simulink model "sim_GPID_LOS"  (R2017a)
settings: Solver=FixedStepAuto  StartTime=0.0  StopTime=inf  FixedStep=0.01  RelTol=1e-3
values from neighbouring files (symbols this model uses):
  trial_params = sim_params(i)    [exec_sim_main.m]
undefined symbols (not defined in the file or in its folder): update_wrap
libraries: simulink x3, emily x1
settings Model: Creator=mitchallain  LastModifiedBy=mitchallain
settings DataIOCC: SaveOutput=off  SaveTime=off

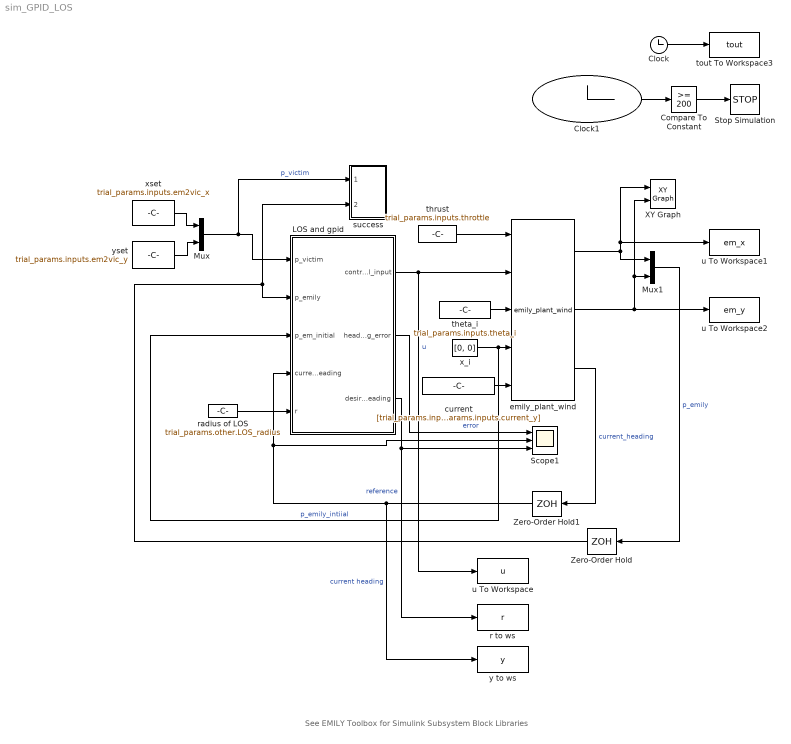
== system sim_GPID_LOS ==
  note: See EMILY Toolbox for Simulink Subsystem Block Libraries
  Clock : Clock
  Clock1 : Clock
  Compare To Constant : simulink/Logic and Bit Operations/Compare To Constant  relop=>=  const=200  OutDataTypeStr=boolean
  LOS and gpid : Subsystem
  Mux : Mux  Inputs=2
  Mux1 : Mux  Inputs=2
  Scope1 : Scope  NumInputPorts=3
  Stop Simulation : Stop
  XY Graph : simulink/Sinks/XY Graph  xmin=-50  xmax=50  ymin=-50  ymax=50  st=-1
  Zero-Order Hold : ZeroOrderHold  SampleTime=0.2
  Zero-Order Hold1 : ZeroOrderHold  SampleTime=0.2
  current : Constant  Value=[trial_params.inputs.current_x, trial_params.inputs.current_y]
  emily_plant_wind : emily/emily_plant_wind
      settings: SourceProductName=EMILY Toolbox
  r to ws : ToWorkspace  VariableName=r  SampleTime=0.2
  radius of LOS : Constant  Value=trial_params.other.LOS_radius
  success : Subsystem  AncestorBlock=emily/success
  theta_i : Constant  Value=trial_params.inputs.theta_i
  thrust : Constant  Value=trial_params.inputs.throttle
  tout To Workspace3 : ToWorkspace  VariableName=tout  SampleTime=0.2
  u To Workspace : ToWorkspace  VariableName=u  SampleTime=0.2
  u To Workspace1 : ToWorkspace  VariableName=em_x  SampleTime=0.2
  u To Workspace2 : ToWorkspace  VariableName=em_y  SampleTime=0.2
  x_i : Constant  Value=[0, 0]
  xset : Constant  Value=trial_params.inputs.em2vic_x
  y to ws : ToWorkspace  VariableName=y  SampleTime=0.2
  yset : Constant  Value=trial_params.inputs.em2vic_y
  wires:
  emily_plant_wind/1 -> XY Graph/1, u To Workspace1/1, Mux1/1
  Mux1/1 -> Zero-Order Hold/1  "p_emily"
  thrust/1 -> emily_plant_wind/1
  Mux/1 -> success/1(p_victim), LOS and gpid/1(p_victim)  "p_victim"
  theta_i/1 -> emily_plant_wind/3
  emily_plant_wind/3 -> Zero-Order Hold1/1  "current_heading"
  xset/1 -> Mux/1
  yset/1 -> Mux/2
  emily_plant_wind/2 -> XY Graph/2, Mux1/2, u To Workspace2/1
  LOS and gpid/2(heading_error) -> Scope1/1  "error"
  LOS and gpid/1(control_input) -> emily_plant_wind/2, u To Workspace/1  "u"
  LOS and gpid/3(desired_heading) -> Scope1/3, r to ws/1  "reference"
  x_i/1 -> LOS and gpid/3(p_em_initial), emily_plant_wind/4  "p_emily_intiial"
  radius of LOS/1 -> LOS and gpid/5(r)
  Zero-Order Hold/1 -> success/2(p_emily), LOS and gpid/2(p_emily)
  Zero-Order Hold1/1 -> y to ws/1, Scope1/2, LOS and gpid/4(current_heading)  "current heading"
  current/1 -> emily_plant_wind/5
  Clock/1 -> tout To Workspace3/1
  Clock1/1 -> Compare To Constant/1
  Compare To Constant/1 -> Stop Simulation/1

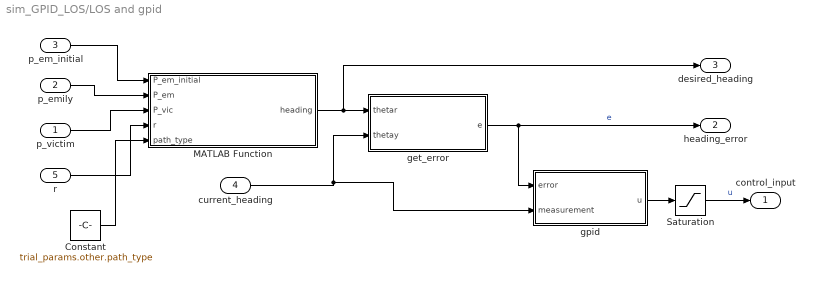
== system sim_GPID_LOS/LOS and gpid ==
  p_victim : Inport
  p_emily : Inport  Port=2
  p_em_initial : Inport  Port=3
  current_heading : Inport  Port=4
  r : Inport  Port=5
  Constant : Constant  Value=trial_params.other.path_type
  MATLAB Function : MATLAB Function  TreatAsAtomicUnit=on
  Saturation : Saturate  UpperLimit=pi/4  LowerLimit=-pi/4
  get_error : MATLAB Function  TreatAsAtomicUnit=on
  gpid : Subsystem
  control_input : Outport
  heading_error : Outport  Port=2
  desired_heading : Outport  Port=3
  wires:
  r/1 -> MATLAB Function/4(r)
  p_em_initial/1 -> MATLAB Function/1(P_em_initial)
  p_emily/1 -> MATLAB Function/2(P_em)
  p_victim/1 -> MATLAB Function/3(P_vic)
  current_heading/1 -> gpid/2(measurement), get_error/2(thetay)
  get_error/1(e) -> gpid/1(error), heading_error/1  "e"
  gpid/1(u) -> Saturation/1
  Saturation/1 -> control_input/1  "u"
  Constant/1 -> MATLAB Function/5(path_type)
  MATLAB Function/1(heading) -> get_error/1(thetar), desired_heading/1

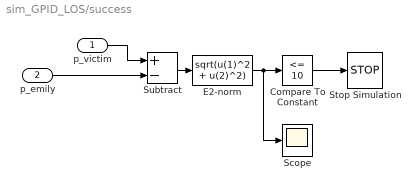
== system sim_GPID_LOS/success ==
  p_victim : Inport
  p_emily : Inport  Port=2
  Compare To Constant : simulink/Logic and Bit Operations/Compare To Constant  relop=<=  const=10  OutDataTypeStr=boolean
  E2-norm : Fcn  Expr=sqrt(u(1)^2 + u(2)^2)
  Scope : Scope
  Stop Simulation : Stop
  Subtract : Sum  Inputs=+-
  wires:
  Subtract/1 -> E2-norm/1
  E2-norm/1 -> Compare To Constant/1, Scope/1
  p_victim/1 -> Subtract/1
  Compare To Constant/1 -> Stop Simulation/1
  p_emily/1 -> Subtract/2

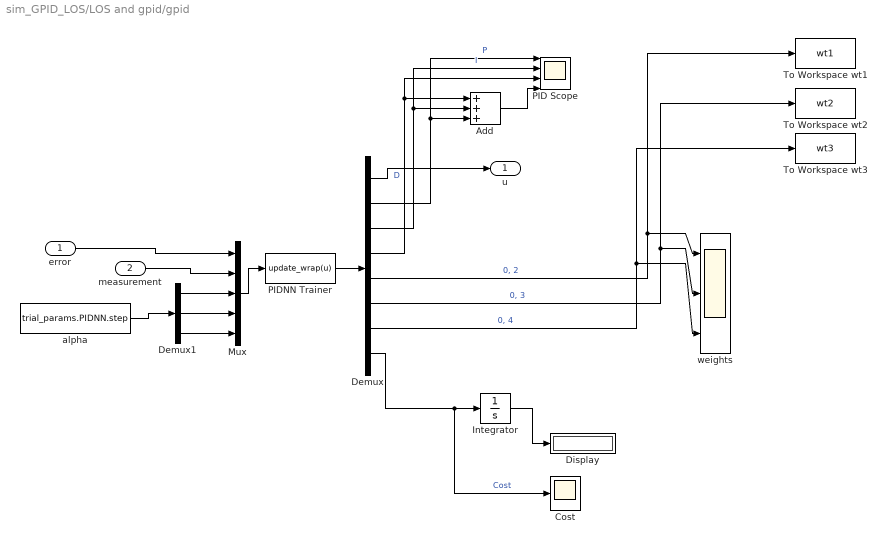
== system sim_GPID_LOS/LOS and gpid/gpid ==
  error : Inport
  measurement : Inport  Port=2
  Add : Sum  Inputs=+++
  Cost : Scope
  Demux : Demux  Outputs=8
  Demux1 : Demux  Outputs=3
  Display : Display
  Integrator : Integrator
  Mux : Mux  Inputs=5
  PID Scope : Scope  NumInputPorts=4
  PIDNN Trainer : MATLABFcn  MATLABFcn=update_wrap(u)  Output1D=off
  To Workspace wt1 : ToWorkspace  VariableName=wt1  SampleTime=-1
  To Workspace wt2 : ToWorkspace  VariableName=wt2  SampleTime=-1
  To Workspace wt3 : ToWorkspace  VariableName=wt3  SampleTime=-1
  alpha : Constant  Value=trial_params.PIDNN.step
  weights : Scope  NumInputPorts=3
  u : Outport
  wires:
  Integrator/1 -> Display/1
  Add/1 -> PID Scope/4
  alpha/1 -> Demux1/1
  Demux/7 -> To Workspace wt3/1, weights/3  "0, 4"
  Demux/6 -> To Workspace wt2/1, weights/2  "0, 3"
  measurement/1 -> Mux/2
  Demux/4 -> PID Scope/3, Add/1  "D"
  Demux/3 -> Add/2, PID Scope/2  "I"
  Mux/1 -> PIDNN Trainer/1
  error/1 -> Mux/1
  Demux/1 -> u/1
  PIDNN Trainer/1 -> Demux/1
  Demux/5 -> To Workspace wt1/1, weights/1  "0, 2"
  Demux/2 -> Add/3, PID Scope/1  "P"
  Demux/8 -> Cost/1, Integrator/1  "Cost"
  Demux1/1 -> Mux/3
  Demux1/2 -> Mux/4
  Demux1/3 -> Mux/5

== matlab function sim_GPID_LOS/LOS and gpid/get_error ==
  data: thetar input; e output; thetay input
function e  = get_error(thetar, thetay)
%UNTITLED Summary of this function goes here
%   FIX THIS MITCH
e = thetar - thetay;
e = mod((e + pi), 2*pi) - pi;
end

== matlab function sim_GPID_LOS/LOS and gpid/MATLAB Function ==
  data: P_em_initial input; heading output; P_em input; P_vic input; r input; path_type input
function heading  = straightpathLOS(P_em_initial, P_em, P_vic, r, path_type)
% This function computes the heading angle according to LOS geometric law
%   Assumes straight line path from initial location to victim
%   If two intersections are produced, the intersection with a higher
%   dispacement parameter (s) is chosen (i.e., farther along path)

% Args:
%   P_em_initial (2-vector): initial (x, y) location of EMILY
%   P_em (2-vector): current (x, y) location of EMILY
%   P_vic (2-vector): victim (x, y) location
%   r (float): radius for LOS control

% Returns:
%   heading: heading unit vector for EMILY in global frame
global trial_params;
% Compute vector from initial EMILY to victim in global frame
P_eiv = P_vic - P_em_initial;

% Compute desired path length and angle
d = norm(P_eiv);
path_angle = atan2(P_eiv(2), P_eiv(1));

% Compute vector from current EMILY to victim
P_ev = P_vic - P_em;

% Bearing is used to seed the fminsearch
bearing = atan2(P_ev(2), P_ev(1));

% Parameterized circle about emily
xLOS = @(phi) P_em(1) + r*cos(phi);
yLOS = @(phi) P_em(2) + r*sin(phi);

switch path_type
    case 1
        x = [P_em_initial(1) P_vic(1)/3  P_vic(1)*2/3  P_vic(1)]; %spline intersection pts
        y = [P_em_initial(2) P_vic(2)*2/3  P_vic(2)*2/3  P_vic(2)];
        pp = spline(x,y);
        path = @(s) ppval(pp,s);
        xy = @(param) (path(param(1)) - xLOS(param(2)))^2 + (path(param(1)) - yLOS(param(2)))^2;
        temp = fminsearch(@(param) xy(param), [P_em(1)+20*cos(bearing), bearing]);
        s_i = temp(1);
        phi_i = temp(2);
        P_es = [s_i - P_em(1); path(s_i) - P_em(2)];
        
    case 2
        x = [P_em_initial(1) P_vic(1)/3 P_vic(1)*2/3 P_vic(1)]; %spline intersection pts
        y = [P_em_initial(2) P_em_initial(2)*4/3 P_vic(2)/3  P_vic(2)];
        pp = spline(x,y);
        path = @(s) ppval(pp,s);
        xy = @(param) (path(param(1)) - xLOS(param(2)))^2 + (path(param(1)) - yLOS(param(2)))^2;
        temp = fminsearch(@(param) xy(param), [P_em(1)+20*cos(bearing), bearing]);
        s_i = temp(1);
        phi_i = temp(2);
        P_es = [s_i - P_em(1); path(s_i) - P_em(2)];
        
    case 3
        x = [P_em_initial(1) P_vic(1)/3 P_vic(1)*2/3 P_vic(1)]; %spline intersection pts
        y = [P_em_initial(2) P_vic(2)*2/3 P_em_initial(2)*4/3  P_vic(2)];
        pp = spline(x,y);
        path = @(s) ppval(pp,s);
        xy = @(param) (path(param(1)) - xLOS(param(2)))^2 + (path(param(1)) - yLOS(param(2)))^2;
        temp = fminsearch(@(param) xy(param), [P_em(1)+20*cos(bearing), bearing]);
        s_i = temp(1);
        phi_i = temp(2);
        P_es = [s_i - P_em(1); path(s_i) - P_em(2)];

    otherwise %'straight'
        xpath = @(s) P_em_initial(1) + s*cos(path_angle);
        ypath = @(s) P_em_initial(2) + s*sin(path_angle);
        xy = @(param) (xpath(param(1)) - xLOS(param(2)))^2 + (ypath(param(1)) - yLOS(param(2)))^2;
        temp = fminsearch(@(param) xy(param), [d, bearing]);
        s_i = min(d, max(0, temp(1)));
        phi_i = temp(2);
        P_es = [xpath(s_i) - P_em(1); ypath(s_i) - P_em(2)];
end
heading = atan2(P_es(2), P_es(1));

% heading = [P_es(1), P_es(2)];
% heading = heading / norm(heading)
end
